simulink model "Coherent_Demodulation"  (R2019b)
settings: Solver=VariableStepAuto  StartTime=0.0  StopTime=0.008  RelTol=1e-3
undefined symbols (not defined in the file): magnitude
libraries: dsparch4 x2
settings Model: Creator=Lenovo  LastModifiedBy=Lenovo

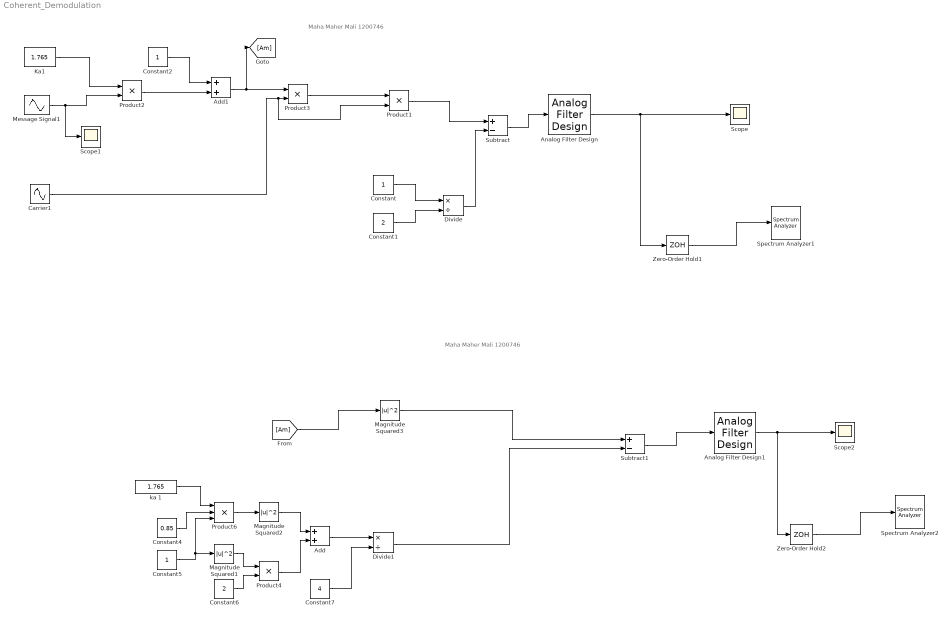
== system Coherent_Demodulation ==
  note: Maha Maher Mali 1200746
  note: Maha Maher Mali 1200746
  Add : Sum
  Add1 : Sum
  Analog Filter Design : dsparch4/Analog Filter Design  method=Butterworth  filttype=Lowpass  N=8  Wlo=2*pi*1000  Whi=80  Rp=2  Rs=40
  Analog Filter Design1 : dsparch4/Analog Filter Design  method=Butterworth  filttype=Lowpass  N=8  Wlo=2*pi*1000  Whi=80  Rp=2  Rs=40
  Carrier1 : Sin  Frequency=2*pi*15000  SampleTime=0
  Constant : Constant
  Constant1 : Constant  Value=2
  Constant2 : Constant
  Constant4 : Constant  Value=0.85
  Constant5 : Constant
  Constant6 : Constant  Value=2
  Constant7 : Constant  Value=4
  Divide : Product  Inputs=*/
  Divide1 : Product  Inputs=*/
  Ka1 : Constant  Value=1.765
  Magnitude Squared1 : Math  Operator=magnitude^2  SignedPower=off  SaturateOnIntegerOverflow=on
  Magnitude Squared2 : Math  Operator=magnitude^2  SignedPower=off  SaturateOnIntegerOverflow=on
  Magnitude Squared3 : Math  Operator=magnitude^2  SignedPower=off  SaturateOnIntegerOverflow=on
  Message Signal1 : Sin  Amplitude=0.85  Frequency=2*pi*1000  SampleTime=0
  Product{1..4} (4 alike) : Product
  Product6 : Product  Inputs=3
  Scope : Scope
  Scope1 : Scope
  Scope2 : Scope
  Spectrum Analyzer1 : SpectrumAnalyzer
  Spectrum Analyzer2 : SpectrumAnalyzer
  Subtract : Sum  Inputs=+-
  Subtract1 : Sum  Inputs=+-
  Zero-Order Hold1 : ZeroOrderHold  SampleTime=1/(10*1e3)
  Zero-Order Hold2 : ZeroOrderHold  SampleTime=1/(10*1e3)
  ka 1 : Constant  Value=1.765
  wires:
  Constant/1 -> Divide/1
  Constant1/1 -> Divide/2
  Divide/1 -> Subtract/2
  Subtract/1 -> Analog Filter Design/1
  Carrier1/1 -> Product1/2, Product3/2
  Ka1/1 -> Product2/1
  Message Signal1/1 -> Scope1/1, Product2/2
  Add1/1 -> [Am], Product3/1
  Constant2/1 -> Add1/1
  Product2/1 -> Add1/2
  Product3/1 -> Product1/1
  Product1/1 -> Subtract/1
  Zero-Order Hold1/1 -> Spectrum Analyzer1/1
  Analog Filter Design/1 -> Zero-Order Hold1/1, Scope/1
  Magnitude Squared3/1 -> Subtract1/1
  Zero-Order Hold2/1 -> Spectrum Analyzer2/1
  Divide1/1 -> Subtract1/2
  Product4/1 -> Add/2
  Analog Filter Design1/1 -> Zero-Order Hold2/1, Scope2/1
  ka 1/1 -> Product6/1
  Constant6/1 -> Product4/2
  Product6/1 -> Magnitude Squared2/1
  Constant4/1 -> Product6/2
  Constant5/1 -> Magnitude Squared1/1, Product6/3
  Constant7/1 -> Divide1/2
  Subtract1/1 -> Analog Filter Design1/1
  Magnitude Squared2/1 -> Add/1
  Magnitude Squared1/1 -> Product4/1
  Add/1 -> Divide1/1
  [Am] -> Magnitude Squared3/1
